simulink model "MAS_CTE"  (R2022b)
settings: Solver=ode4  StartTime=0.0  StopTime=30  FixedStep=0.01  RelTol=1e-3
(part 1 of 3)
settings Model: Creator=a1752760  LastModifiedBy=yfeih
settings SolverCC: AlgebraicLoopSolver=TrustRegion
settings DebuggingCC: UnconnectedInputMsg=warning  UnconnectedOutputMsg=warning  UnconnectedLineMsg=warning  SFMachineParentedDataDiag=warning
settings ModelReferenceCC: EnableRefExpFcnMdlSchedulingChecks=on
settings RTWCC: DLArmComputeVersion=19.05

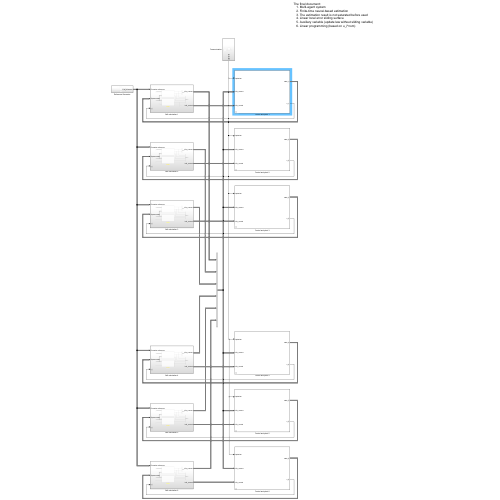
[thumbnail: Simulink's stored preview of the top-level diagram]
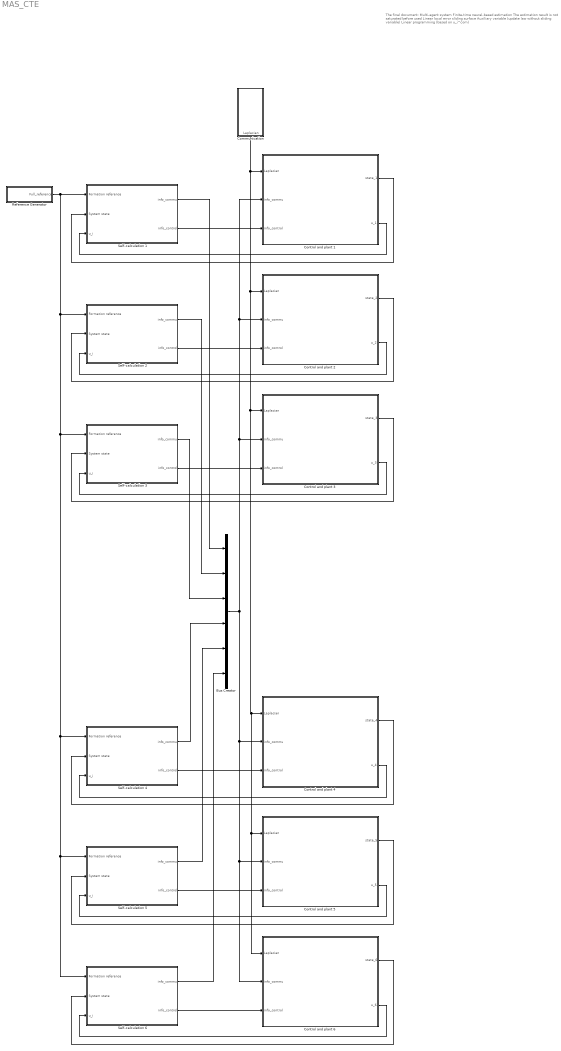
== system MAS_CTE ==
  note: The final document:
      | Multi-agent system
      | Finite-time neural-based estimation
      | The estimation result is not saturated before used
      | Linear local error sliding surface
      | Auxiliary variable (update law without sliding variable)
      | Linear programming (based on u_i^com)
  Bus Creator : BusCreator  Inputs=6
  Communication : Subsystem
  Control and plant 1 : Subsystem  mask{x_1=[3.5;1.5;pi/5], UpperLimit=0.2, LowerLimit=-0.2}
      mask prompts: x_1 "Simulink:blkprm_prompts:IntegratorInitCond"; UpperLimit "Simulink:blkprm_prompts:SaturateUpLim"; LowerLimit "Simulink:blkprm_prompts:SaturateLowLim"
      mask TypeOptions x_1: x_1/InitialCondition
      mask TypeOptions UpperLimit: Saturation/UpperLimit
      mask TypeOptions LowerLimit: Saturation/LowerLimit
      mask DialogControl x_1 Prompt: 初始条件:
      mask DialogControl UpperLimit Prompt: 上限:
      mask DialogControl LowerLimit Prompt: 下限:
  Control and plant 2 : Subsystem  mask{x_2=[-1.8;2.2;-pi/4], UpperLimit=0.2, LowerLimit=-0.2}
      mask prompts: x_2 "Simulink:blkprm_prompts:IntegratorInitCond"; UpperLimit "Simulink:blkprm_prompts:SaturateUpLim"; LowerLimit "Simulink:blkprm_prompts:SaturateLowLim"
      mask TypeOptions x_2: x_2/InitialCondition
      mask TypeOptions UpperLimit: Saturation/UpperLimit
      mask TypeOptions LowerLimit: Saturation/LowerLimit
      mask DialogControl x_2 Prompt: 初始条件:
      mask DialogControl UpperLimit Prompt: 上限:
      mask DialogControl LowerLimit Prompt: 下限:
  Control and plant 3 : Subsystem  mask{x_3=[-0.5;0.2;pi/6], UpperLimit=0.2, LowerLimit=-0.2}
      mask prompts: x_3 "Simulink:blkprm_prompts:IntegratorInitCond"; UpperLimit "Simulink:blkprm_prompts:SaturateUpLim"; LowerLimit "Simulink:blkprm_prompts:SaturateLowLim"
      mask TypeOptions x_3: x_3/InitialCondition
      mask TypeOptions UpperLimit: Saturation/UpperLimit
      mask TypeOptions LowerLimit: Saturation/LowerLimit
      mask DialogControl x_3 Prompt: 初始条件:
      mask DialogControl UpperLimit Prompt: 上限:
      mask DialogControl LowerLimit Prompt: 下限:
  Control and plant 4 : Subsystem  mask{x_4=[-1;-1.8;pi/4], UpperLimit=0.2, LowerLimit=-0.2}
      mask prompts: x_4 "Simulink:blkprm_prompts:IntegratorInitCond"; UpperLimit "Simulink:blkprm_prompts:SaturateUpLim"; LowerLimit "Simulink:blkprm_prompts:SaturateLowLim"
      mask TypeOptions x_4: x_4/InitialCondition
      mask TypeOptions UpperLimit: Saturation/UpperLimit
      mask TypeOptions LowerLimit: Saturation/LowerLimit
      mask DialogControl x_4 Prompt: 初始条件:
      mask DialogControl UpperLimit Prompt: 上限:
      mask DialogControl LowerLimit Prompt: 下限:
  Control and plant 5 : Subsystem  mask{x_5=[0.2;-1.8;-pi/4], UpperLimit=0.2, LowerLimit=-0.2}
      mask prompts: x_5 "Simulink:blkprm_prompts:IntegratorInitCond"; UpperLimit "Simulink:blkprm_prompts:SaturateUpLim"; LowerLimit "Simulink:blkprm_prompts:SaturateLowLim"
      mask TypeOptions x_5: x_5/InitialCondition
      mask TypeOptions UpperLimit: Saturation/UpperLimit
      mask TypeOptions LowerLimit: Saturation/LowerLimit
      mask DialogControl x_5 Prompt: 初始条件:
      mask DialogControl UpperLimit Prompt: 上限:
      mask DialogControl LowerLimit Prompt: 下限:
  Control and plant 6 : Subsystem  mask{x_6=[1.2;-0.8;pi/6], UpperLimit=0.2, LowerLimit=-0.2}
      mask prompts: x_6 "Simulink:blkprm_prompts:IntegratorInitCond"; UpperLimit "Simulink:blkprm_prompts:SaturateUpLim"; LowerLimit "Simulink:blkprm_prompts:SaturateLowLim"
      mask TypeOptions x_6: x_6/InitialCondition
      mask TypeOptions UpperLimit: Saturation/UpperLimit
      mask TypeOptions LowerLimit: Saturation/LowerLimit
      mask DialogControl x_6 Prompt: 初始条件:
      mask DialogControl UpperLimit Prompt: 上限:
      mask DialogControl LowerLimit Prompt: 下限:
  Reference Generator : Subsystem
  Self-calculation 1 : Subsystem
  Self-calculation 2 : Subsystem
  Self-calculation 3 : Subsystem
  Self-calculation 4 : Subsystem
  Self-calculation 5 : Subsystem
  Self-calculation 6 : Subsystem
  wires:
  Control and plant 1/1(state_1) -> Self-calculation 1/2(System state)
  Control and plant 1/2(u_1) -> Self-calculation 1/3(u_i)
  Self-calculation 1/2(info_control) -> Control and plant 1/3(info_control)
  Communication/1(Laplacian) -> Control and plant 2/1(Laplacian), Control and plant 3/1(Laplacian), Control and plant 4/1(Laplacian), Control and plant 6/1(Laplacian), Control and plant 5/1(Laplacian), Control and plant 1/1(Laplacian)
  Self-calculation 2/2(info_control) -> Control and plant 2/3(info_control)
  Control and plant 2/1(state_2) -> Self-calculation 2/2(System state)
  Control and plant 2/2(u_2) -> Self-calculation 2/3(u_i)
  Self-calculation 3/2(info_control) -> Control and plant 3/3(info_control)
  Control and plant 3/1(state_3) -> Self-calculation 3/2(System state)
  Control and plant 3/2(u_3) -> Self-calculation 3/3(u_i)
  Self-calculation 4/2(info_control) -> Control and plant 4/3(info_control)
  Control and plant 4/1(state_4) -> Self-calculation 4/2(System state)
  Control and plant 4/2(u_4) -> Self-calculation 4/3(u_i)
  Control and plant 5/1(state_5) -> Self-calculation 5/2(System state)
  Control and plant 5/2(u_5) -> Self-calculation 5/3(u_i)
  Control and plant 6/2(u_6) -> Self-calculation 6/3(u_i)
  Reference Generator/1(Full_reference) -> Self-calculation 6/1(Formation reference), Self-calculation 5/1(Formation reference), Self-calculation 4/1(Formation reference), Self-calculation 3/1(Formation reference), Self-calculation 2/1(Formation reference), Self-calculation 1/1(Formation reference)
  Control and plant 6/1(state_6) -> Self-calculation 6/2(System state)
  Self-calculation 5/2(info_control) -> Control and plant 5/3(info_control)
  Self-calculation 6/2(info_control) -> Control and plant 6/3(info_control)
  Self-calculation 1/1(info_commu) -> Bus Creator/1
  Self-calculation 2/1(info_commu) -> Bus Creator/2
  Self-calculation 3/1(info_commu) -> Bus Creator/3
  Self-calculation 4/1(info_commu) -> Bus Creator/4
  Self-calculation 5/1(info_commu) -> Bus Creator/5
  Self-calculation 6/1(info_commu) -> Bus Creator/6
  Bus Creator/1 -> Control and plant 3/2(info_commu), Control and plant 2/2(info_commu), Control and plant 1/2(info_commu), Control and plant 4/2(info_commu), Control and plant 6/2(info_commu), Control and plant 5/2(info_commu)

== system MAS_CTE/Communication ==
  Add : Sum
  Communication Topology : Constant  Value=[3,-1,0,0,-1,-1;0,1,-1,0,0,0;0,-1,2,-1,0,0;0,0,-1,2,-1,0;-1,0,0,0,1,0;0,0,0,0,-1,1]  VectorParams1D=off
  Constant : Constant  Value=2  VectorParams1D=off
  Product : Product
  Reference Feeding : Constant  Value=[1,0,0,0,0,0;0,1,0,0,0,0;0,0,1,0,0,0;0,0,0,1,0,0;0,0,0,0,1,0;0,0,0,0,0,1]  VectorParams1D=off
  Laplacian : Outport  VectorParamsAs1DForOutWhenUnconnected=off
  wires:
  Constant/1 -> Product/2
  Reference Feeding/1 -> Product/1
  Communication Topology/1 -> Add/1
  Product/1 -> Add/2
  Add/1 -> Laplacian/1

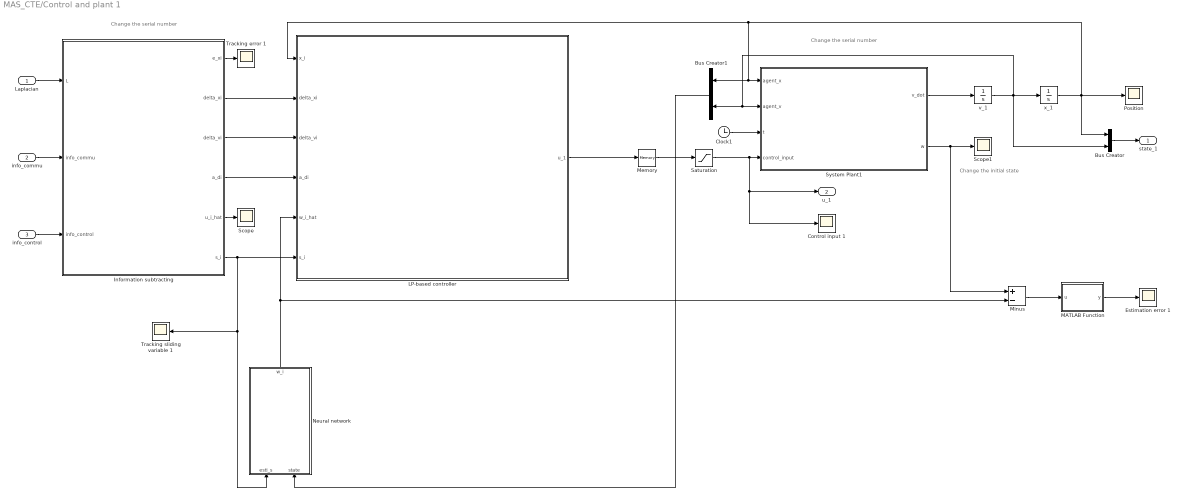
== system MAS_CTE/Control and plant 1 ==
  note: Change the serial number
  note: Change the serial number
  note: Change the initial state
  Laplacian : Inport
  info_commu : Inport  Port=2
  info_control : Inport  Port=3
  Bus Creator : BusCreator  Inputs=2
  Bus Creator1 : BusCreator  Inputs=2
  Clock1 : Clock
  Control input 1 : Scope
  Estimation error 1 : Scope
  Information subtracting : MATLAB Function  TreatAsAtomicUnit=on
  LP-based controller : Subsystem
  MATLAB Function : MATLAB Function  TreatAsAtomicUnit=on
  Memory : Memory  InitialCondition=[0;0;0]
  Minus : Sum  Inputs=+-
  Neural network : Subsystem
  Position : Scope
  Saturation : Saturate  UpperLimit=UpperLimit  LowerLimit=LowerLimit
  Scope : Scope
  Scope1 : Scope
  System Plant1 : MATLAB Function  TreatAsAtomicUnit=on
  Tracking error 1 : Scope
  Tracking sliding variable 1 : Scope
  v_1 : Integrator  InitialCondition=[0;0;0]  ContinuousStateAttributes='speed'
  x_1 : Integrator  Tag=Position_x1  InitialCondition=x_1  ContinuousStateAttributes='position'
  state_1 : Outport
  u_1 : Outport  Port=2
  wires:
  Clock1/1 -> System Plant1/3(t)
  System Plant1/1(v_dot) -> v_1/1
  v_1/1 -> Bus Creator/2, x_1/1, System Plant1/2(agent_v), Bus Creator1/2
  x_1/1 -> Bus Creator/1, Position/1, LP-based controller/1(x_i), System Plant1/1(agent_x), Bus Creator1/1
  System Plant1/2(w) -> Minus/1, Scope1/1
  Bus Creator/1 -> state_1/1
  info_commu/1 -> Information subtracting/2(info_commu)
  info_control/1 -> Information subtracting/3(info_control)
  Laplacian/1 -> Information subtracting/1(L)
  MATLAB Function/1(y) -> Estimation error 1/1
  Minus/1 -> MATLAB Function/1(u)
  Saturation/1 -> u_1/1, Control input 1/1, System Plant1/4(control_input)
  Memory/1 -> Saturation/1
  Information subtracting/1(e_xi) -> Tracking error 1/1
  LP-based controller/1(u_1) -> Memory/1
  Information subtracting/6(s_i) -> Tracking sliding variable 1/1, Neural network/1(esti_s), LP-based controller/6(s_i)
  Information subtracting/4(a_di) -> LP-based controller/4(a_di)
  Information subtracting/3(delta_vi) -> LP-based controller/3(delta_vi)
  Information subtracting/2(delta_xi) -> LP-based controller/2(delta_xi)
  Bus Creator1/1 -> Neural network/2(state)
  Information subtracting/5(u_i_hat) -> Scope/1
  Neural network/1(w_i) -> LP-based controller/5(w_i_hat), Minus/2

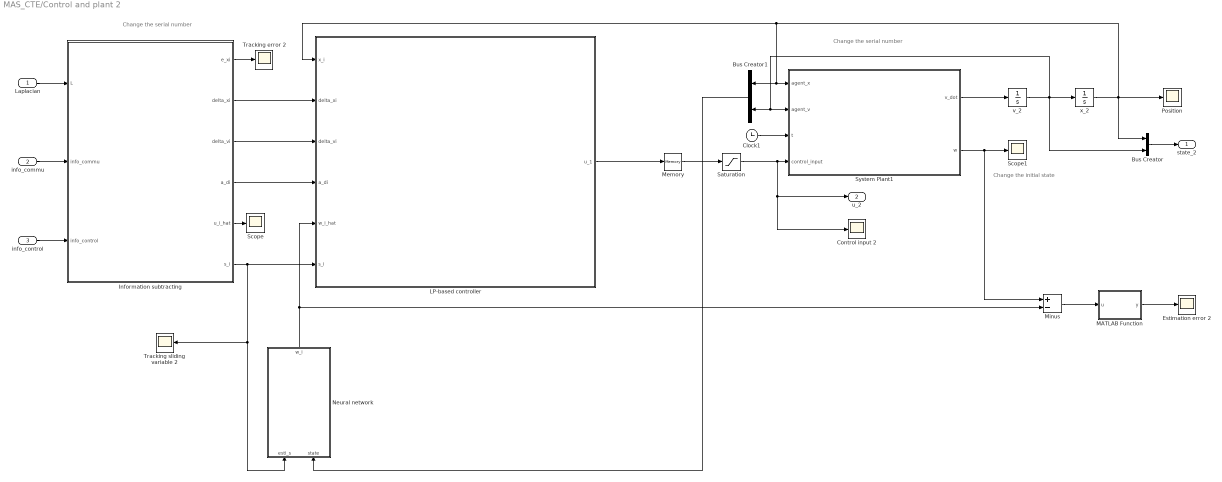
== system MAS_CTE/Control and plant 2 ==
  note: Change the serial number
  note: Change the serial number
  note: Change the initial state
  Laplacian : Inport
  info_commu : Inport  Port=2
  info_control : Inport  Port=3
  Bus Creator : BusCreator  Inputs=2
  Bus Creator1 : BusCreator  Inputs=2
  Clock1 : Clock
  Control input 2 : Scope
  Estimation error 2 : Scope
  Information subtracting : MATLAB Function  TreatAsAtomicUnit=on
  LP-based controller : Subsystem
  MATLAB Function : MATLAB Function  TreatAsAtomicUnit=on
  Memory : Memory  InitialCondition=[0;0;0]
  Minus : Sum  Inputs=+-
  Neural network : Subsystem
  Position : Scope
  Saturation : Saturate  UpperLimit=UpperLimit  LowerLimit=LowerLimit
  Scope : Scope
  Scope1 : Scope
  System Plant1 : MATLAB Function  TreatAsAtomicUnit=on
  Tracking error 2 : Scope
  Tracking sliding variable 2 : Scope
  v_2 : Integrator  InitialCondition=[0;0;0]  ContinuousStateAttributes='speed'
  x_2 : Integrator  Tag=Position_x1  InitialCondition=x_2  ContinuousStateAttributes='position'
  state_2 : Outport
  u_2 : Outport  Port=2
  wires:
  Clock1/1 -> System Plant1/3(t)
  System Plant1/1(v_dot) -> v_2/1
  v_2/1 -> Bus Creator/2, x_2/1, System Plant1/2(agent_v), Bus Creator1/2
  x_2/1 -> Bus Creator/1, Position/1, LP-based controller/1(x_i), System Plant1/1(agent_x), Bus Creator1/1
  System Plant1/2(w) -> Minus/1, Scope1/1
  Bus Creator/1 -> state_2/1
  info_commu/1 -> Information subtracting/2(info_commu)
  info_control/1 -> Information subtracting/3(info_control)
  Laplacian/1 -> Information subtracting/1(L)
  MATLAB Function/1(y) -> Estimation error 2/1
  Minus/1 -> MATLAB Function/1(u)
  Saturation/1 -> u_2/1, Control input 2/1, System Plant1/4(control_input)
  Memory/1 -> Saturation/1
  Information subtracting/1(e_xi) -> Tracking error 2/1
  LP-based controller/1(u_1) -> Memory/1
  Information subtracting/2(delta_xi) -> LP-based controller/2(delta_xi)
  Information subtracting/3(delta_vi) -> LP-based controller/3(delta_vi)
  Information subtracting/4(a_di) -> LP-based controller/4(a_di)
  Information subtracting/6(s_i) -> Tracking sliding variable 2/1, Neural network/1(esti_s), LP-based controller/6(s_i)
  Bus Creator1/1 -> Neural network/2(state)
  Information subtracting/5(u_i_hat) -> Scope/1
  Neural network/1(w_i) -> Minus/2, LP-based controller/5(w_i_hat)

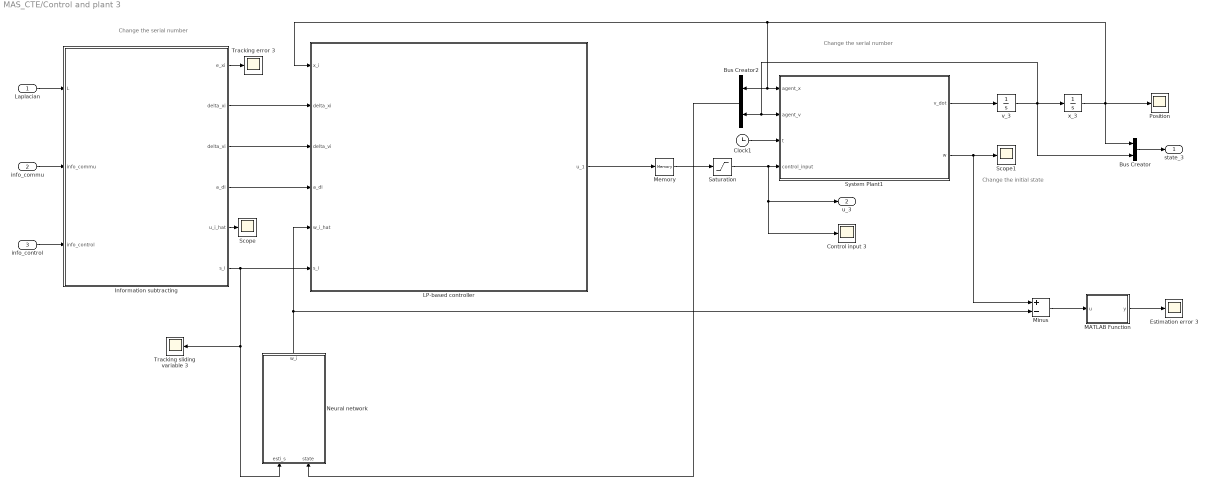
== system MAS_CTE/Control and plant 3 ==
  note: Change the serial number
  note: Change the serial number
  note: Change the initial state
  Laplacian : Inport
  info_commu : Inport  Port=2
  info_control : Inport  Port=3
  Bus Creator : BusCreator  Inputs=2
  Bus Creator2 : BusCreator  Inputs=2
  Clock1 : Clock
  Control input 3 : Scope
  Estimation error 3 : Scope
  Information subtracting : MATLAB Function  TreatAsAtomicUnit=on
  LP-based controller : Subsystem
  MATLAB Function : MATLAB Function  TreatAsAtomicUnit=on
  Memory : Memory  InitialCondition=[0;0;0]
  Minus : Sum  Inputs=+-
  Neural network : Subsystem
  Position : Scope
  Saturation : Saturate  UpperLimit=UpperLimit  LowerLimit=LowerLimit
  Scope : Scope
  Scope1 : Scope
  System Plant1 : MATLAB Function  TreatAsAtomicUnit=on
  Tracking error 3 : Scope
  Tracking sliding variable 3 : Scope
  v_3 : Integrator  InitialCondition=[0;0;0]  ContinuousStateAttributes='speed'
  x_3 : Integrator  Tag=Position_x1  InitialCondition=x_3  ContinuousStateAttributes='position'
  state_3 : Outport
  u_3 : Outport  Port=2
  wires:
  Clock1/1 -> System Plant1/3(t)
  System Plant1/1(v_dot) -> v_3/1
  v_3/1 -> Bus Creator/2, x_3/1, Bus Creator2/2, System Plant1/2(agent_v)
  x_3/1 -> Bus Creator/1, Position/1, LP-based controller/1(x_i), System Plant1/1(agent_x), Bus Creator2/1
  System Plant1/2(w) -> Minus/1, Scope1/1
  Bus Creator/1 -> state_3/1
  info_commu/1 -> Information subtracting/2(info_commu)
  info_control/1 -> Information subtracting/3(info_control)
  Laplacian/1 -> Information subtracting/1(L)
  MATLAB Function/1(y) -> Estimation error 3/1
  Minus/1 -> MATLAB Function/1(u)
  Saturation/1 -> u_3/1, Control input 3/1, System Plant1/4(control_input)
  Memory/1 -> Saturation/1
  Information subtracting/1(e_xi) -> Tracking error 3/1
  LP-based controller/1(u_1) -> Memory/1
  Information subtracting/4(a_di) -> LP-based controller/4(a_di)
  Information subtracting/3(delta_vi) -> LP-based controller/3(delta_vi)
  Information subtracting/2(delta_xi) -> LP-based controller/2(delta_xi)
  Information subtracting/5(u_i_hat) -> Scope/1
  Information subtracting/6(s_i) -> Tracking sliding variable 3/1, Neural network/1(esti_s), LP-based controller/6(s_i)
  Bus Creator2/1 -> Neural network/2(state)
  Neural network/1(w_i) -> LP-based controller/5(w_i_hat), Minus/2

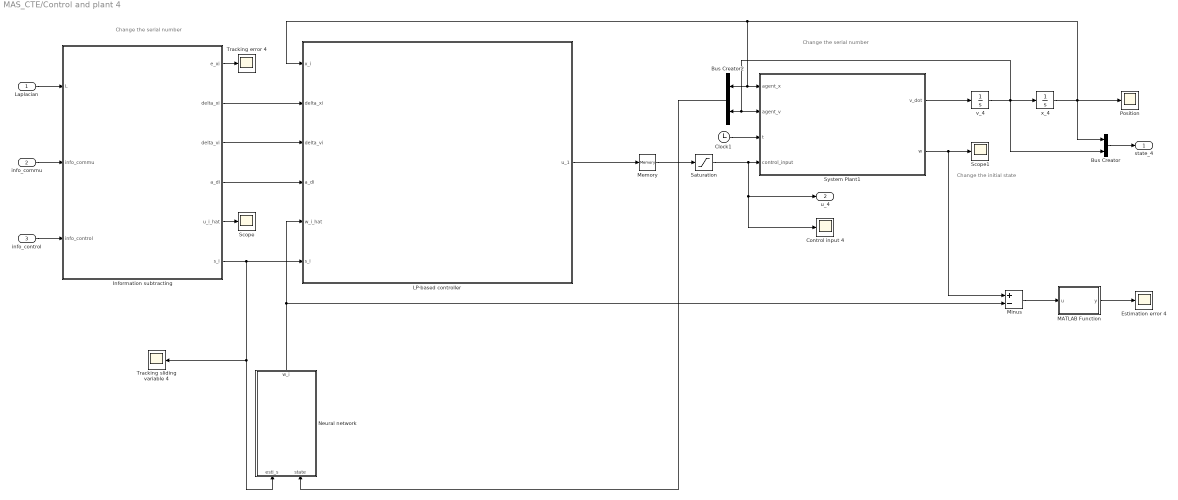
== system MAS_CTE/Control and plant 4 ==
  note: Change the serial number
  note: Change the serial number
  note: Change the initial state
  Laplacian : Inport
  info_commu : Inport  Port=2
  info_control : Inport  Port=3
  Bus Creator : BusCreator  Inputs=2
  Bus Creator2 : BusCreator  Inputs=2
  Clock1 : Clock
  Control input 4 : Scope
  Estimation error 4 : Scope
  Information subtracting : MATLAB Function  TreatAsAtomicUnit=on
  LP-based controller : Subsystem
  MATLAB Function : MATLAB Function  TreatAsAtomicUnit=on
  Memory : Memory  InitialCondition=[0;0;0]
  Minus : Sum  Inputs=+-
  Neural network : Subsystem
  Position : Scope
  Saturation : Saturate  UpperLimit=UpperLimit  LowerLimit=LowerLimit
  Scope : Scope
  Scope1 : Scope
  System Plant1 : MATLAB Function  TreatAsAtomicUnit=on
  Tracking error 4 : Scope
  Tracking sliding variable 4 : Scope
  v_4 : Integrator  InitialCondition=[0;0;0]  ContinuousStateAttributes='speed'
  x_4 : Integrator  Tag=Position_x1  InitialCondition=x_4  ContinuousStateAttributes='position'
  state_4 : Outport
  u_4 : Outport  Port=2
  wires:
  Clock1/1 -> System Plant1/3(t)
  System Plant1/1(v_dot) -> v_4/1
  v_4/1 -> Bus Creator/2, x_4/1, System Plant1/2(agent_v), Bus Creator2/2
  x_4/1 -> Bus Creator/1, Position/1, LP-based controller/1(x_i), System Plant1/1(agent_x), Bus Creator2/1
  System Plant1/2(w) -> Minus/1, Scope1/1
  Bus Creator/1 -> state_4/1
  info_commu/1 -> Information subtracting/2(info_commu)
  info_control/1 -> Information subtracting/3(info_control)
  Laplacian/1 -> Information subtracting/1(L)
  MATLAB Function/1(y) -> Estimation error 4/1
  Minus/1 -> MATLAB Function/1(u)
  Saturation/1 -> u_4/1, Control input 4/1, System Plant1/4(control_input)
  Memory/1 -> Saturation/1
  Information subtracting/1(e_xi) -> Tracking error 4/1
  LP-based controller/1(u_1) -> Memory/1
  Information subtracting/3(delta_vi) -> LP-based controller/3(delta_vi)
  Information subtracting/2(delta_xi) -> LP-based controller/2(delta_xi)
  Information subtracting/4(a_di) -> LP-based controller/4(a_di)
  Information subtracting/6(s_i) -> Tracking sliding variable 4/1, Neural network/1(esti_s), LP-based controller/6(s_i)
  Bus Creator2/1 -> Neural network/2(state)
  Neural network/1(w_i) -> Minus/2, LP-based controller/5(w_i_hat)
  Information subtracting/5(u_i_hat) -> Scope/1

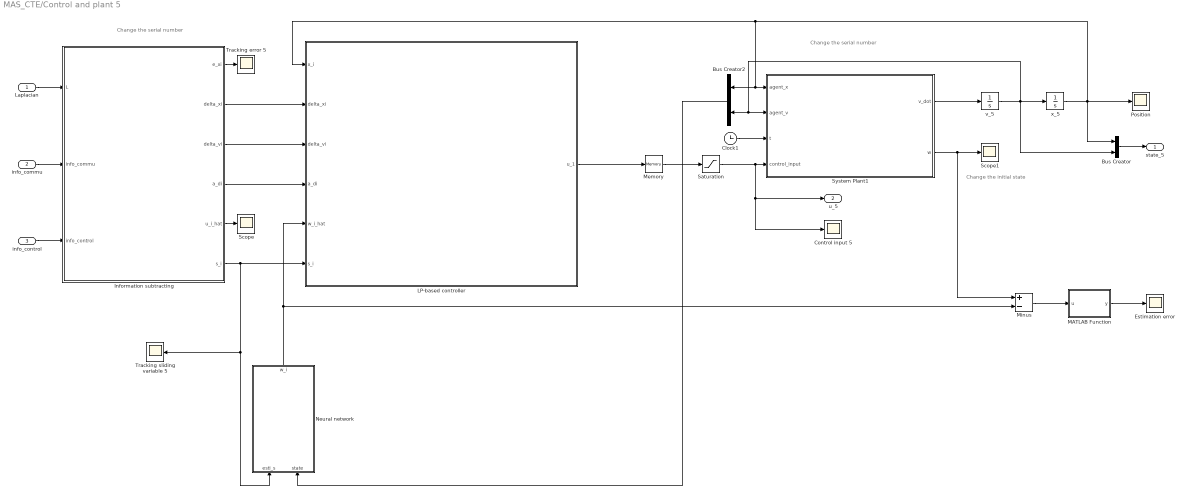
== system MAS_CTE/Control and plant 5 ==
  note: Change the serial number
  note: Change the serial number
  note: Change the initial state
  Laplacian : Inport
  info_commu : Inport  Port=2
  info_control : Inport  Port=3
  Bus Creator : BusCreator  Inputs=2
  Bus Creator2 : BusCreator  Inputs=2
  Clock1 : Clock
  Control input 5 : Scope
  Estimation error : Scope
  Information subtracting : MATLAB Function  TreatAsAtomicUnit=on
  LP-based controller : Subsystem
  MATLAB Function : MATLAB Function  TreatAsAtomicUnit=on
  Memory : Memory  InitialCondition=[0;0;0]
  Minus : Sum  Inputs=+-
  Neural network : Subsystem
  Position : Scope
  Saturation : Saturate  UpperLimit=UpperLimit  LowerLimit=LowerLimit
  Scope : Scope
  Scope1 : Scope
  System Plant1 : MATLAB Function  TreatAsAtomicUnit=on
  Tracking error 5 : Scope
  Tracking sliding variable 5 : Scope
  v_5 : Integrator  InitialCondition=[0;0;0]  ContinuousStateAttributes='speed'
  x_5 : Integrator  Tag=Position_x1  InitialCondition=x_5  ContinuousStateAttributes='position'
  state_5 : Outport
  u_5 : Outport  Port=2
  wires:
  Clock1/1 -> System Plant1/3(t)
  System Plant1/1(v_dot) -> v_5/1
  v_5/1 -> Bus Creator/2, x_5/1, System Plant1/2(agent_v), Bus Creator2/2
  x_5/1 -> Bus Creator/1, Position/1, LP-based controller/1(x_i), Bus Creator2/1, System Plant1/1(agent_x)
  System Plant1/2(w) -> Minus/1, Scope1/1
  Bus Creator/1 -> state_5/1
  info_commu/1 -> Information subtracting/2(info_commu)
  info_control/1 -> Information subtracting/3(info_control)
  Laplacian/1 -> Information subtracting/1(L)
  MATLAB Function/1(y) -> Estimation error/1
  Minus/1 -> MATLAB Function/1(u)
  Saturation/1 -> u_5/1, Control input 5/1, System Plant1/4(control_input)
  Memory/1 -> Saturation/1
  Information subtracting/1(e_xi) -> Tracking error 5/1
  LP-based controller/1(u_1) -> Memory/1
  Information subtracting/3(delta_vi) -> LP-based controller/3(delta_vi)
  Information subtracting/2(delta_xi) -> LP-based controller/2(delta_xi)
  Information subtracting/4(a_di) -> LP-based controller/4(a_di)
  Information subtracting/6(s_i) -> Tracking sliding variable 5/1, Neural network/1(esti_s), LP-based controller/6(s_i)
  Bus Creator2/1 -> Neural network/2(state)
  Information subtracting/5(u_i_hat) -> Scope/1
  Neural network/1(w_i) -> Minus/2, LP-based controller/5(w_i_hat)

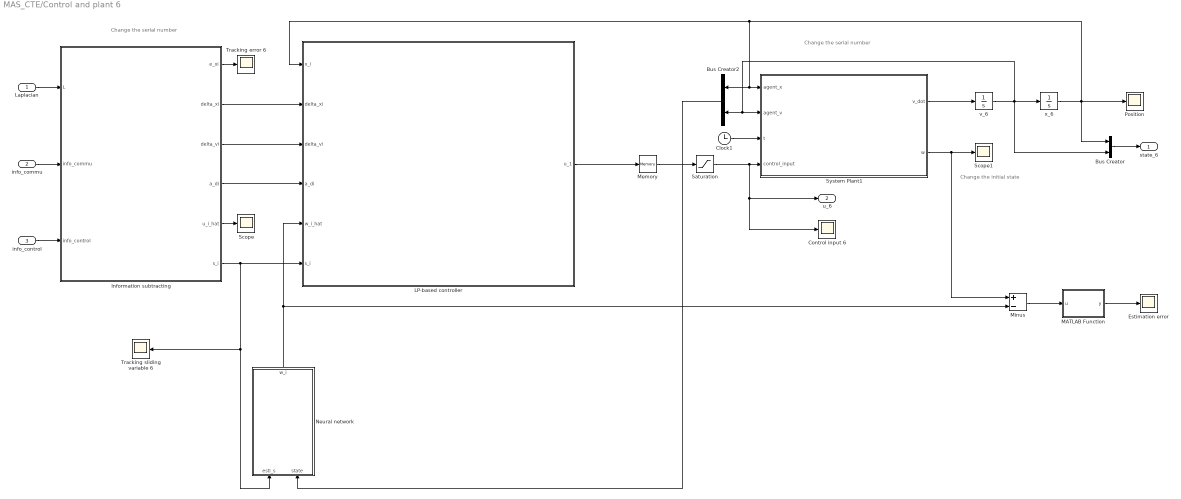
== system MAS_CTE/Control and plant 6 ==
  note: Change the serial number
  note: Change the serial number
  note: Change the initial state
  Laplacian : Inport
  info_commu : Inport  Port=2
  info_control : Inport  Port=3
  Bus Creator : BusCreator  Inputs=2
  Bus Creator2 : BusCreator  Inputs=2
  Clock1 : Clock
  Control input 6 : Scope
  Estimation error : Scope
  Information subtracting : MATLAB Function  TreatAsAtomicUnit=on
  LP-based controller : Subsystem
  MATLAB Function : MATLAB Function  TreatAsAtomicUnit=on
  Memory : Memory  InitialCondition=[0;0;0]
  Minus : Sum  Inputs=+-
  Neural network : Subsystem
  Position : Scope
  Saturation : Saturate  UpperLimit=UpperLimit  LowerLimit=LowerLimit
  Scope : Scope
  Scope1 : Scope
  System Plant1 : MATLAB Function  TreatAsAtomicUnit=on
  Tracking error 6 : Scope
  Tracking sliding variable 6 : Scope
  v_6 : Integrator  InitialCondition=[0;0;0]  ContinuousStateAttributes='speed'
  x_6 : Integrator  Tag=Position_x1  InitialCondition=x_6  ContinuousStateAttributes='position'
  state_6 : Outport
  u_6 : Outport  Port=2
  wires:
  Clock1/1 -> System Plant1/3(t)
  System Plant1/1(v_dot) -> v_6/1
  v_6/1 -> Bus Creator/2, x_6/1, System Plant1/2(agent_v), Bus Creator2/2
  x_6/1 -> Bus Creator/1, Position/1, LP-based controller/1(x_i), System Plant1/1(agent_x), Bus Creator2/1
  System Plant1/2(w) -> Minus/1, Scope1/1
  Bus Creator/1 -> state_6/1
  info_commu/1 -> Information subtracting/2(info_commu)
  info_control/1 -> Information subtracting/3(info_control)
  Laplacian/1 -> Information subtracting/1(L)
  MATLAB Function/1(y) -> Estimation error/1
  Minus/1 -> MATLAB Function/1(u)
  Saturation/1 -> u_6/1, Control input 6/1, System Plant1/4(control_input)
  Memory/1 -> Saturation/1
  Information subtracting/1(e_xi) -> Tracking error 6/1
  LP-based controller/1(u_1) -> Memory/1
  Information subtracting/2(delta_xi) -> LP-based controller/2(delta_xi)
  Information subtracting/3(delta_vi) -> LP-based controller/3(delta_vi)
  Information subtracting/4(a_di) -> LP-based controller/4(a_di)
  Information subtracting/6(s_i) -> Tracking sliding variable 6/1, Neural network/1(esti_s), LP-based controller/6(s_i)
  Bus Creator2/1 -> Neural network/2(state)
  Neural network/1(w_i) -> Minus/2, LP-based controller/5(w_i_hat)
  Information subtracting/5(u_i_hat) -> Scope/1

== system MAS_CTE/Reference Generator ==
  Acceleration Reference : MATLAB Function  TreatAsAtomicUnit=on
  Bus Creator : BusCreator  Inputs=3
  Centre acceleration : Scope
  Centre position : Scope
  Centre velocity : Scope
  Clock : Clock
  Position Reference : MATLAB Function  TreatAsAtomicUnit=on
  Position_ref : Scope
  Velocity Reference : MATLAB Function  TreatAsAtomicUnit=on
  Full_reference : Outport  VectorParamsAs1DForOutWhenUnconnected=off
  wires:
  Clock/1 -> Velocity Reference/1(t), Acceleration Reference/1(t), Position Reference/1(t)
  Position Reference/1(x_d) -> Bus Creator/1, Position_ref/1
  Position Reference/2(centre) -> Centre position/1
  Velocity Reference/2(centre) -> Centre velocity/1
  Acceleration Reference/2(centre) -> Centre acceleration/1
  Velocity Reference/1(v_d) -> Bus Creator/2
  Acceleration Reference/1(a_d) -> Bus Creator/3
  Bus Creator/1 -> Full_reference/1

== system MAS_CTE/Self-calculation 1 ==
  note: Change the serial number
  Formation reference : Inport
  System state : Inport  Port=2
  u_i : Inport  Port=3
  Bus Creator : BusCreator  Inputs=4
  Bus Creator1 : BusCreator  Inputs=2
  E_1 : Scope
  Observer : Subsystem  mask{InitialCondition=[3.5;1.5;pi/5]}
      mask prompts: InitialCondition "Simulink:blkprm_prompts:IntegratorInitCond"
      mask TypeOptions InitialCondition: virtual_pos/InitialCondition
      mask DialogControl InitialCondition Prompt: 初始条件:
  Tracking error calculation : Subsystem
  info_commu : Outport
  info_control : Outport  Port=2
  wires:
  Formation reference/1 -> Tracking error calculation/1(ref)
  System state/1 -> Tracking error calculation/2(state), Observer/1(state)
  Tracking error calculation/1(delta_xi) -> Bus Creator/1, Bus Creator1/1
  Tracking error calculation/2(delta_vi) -> Bus Creator/2, Bus Creator1/2
  Tracking error calculation/3(a_d) -> Bus Creator/3
  Bus Creator1/1 -> info_commu/1
  Bus Creator/1 -> info_control/1
  u_i/1 -> Observer/2(u_i)
  Observer/1(E_i) -> E_1/1, Bus Creator/4

== system MAS_CTE/Self-calculation 2 ==
  note: Change the serial number
  Formation reference : Inport
  System state : Inport  Port=2
  u_i : Inport  Port=3
  Bus Creator : BusCreator  Inputs=4
  Bus Creator1 : BusCreator  Inputs=2
  Observer : Subsystem  mask{InitialCondition=[-1.8;2.2;-pi/4]}
      mask prompts: InitialCondition "Simulink:blkprm_prompts:IntegratorInitCond"
      mask TypeOptions InitialCondition: virtual_pos/InitialCondition
      mask DialogControl InitialCondition Prompt: 初始条件:
  Tracking error calculation : Subsystem
  info_commu : Outport
  info_control : Outport  Port=2
  wires:
  Formation reference/1 -> Tracking error calculation/1(ref)
  System state/1 -> Observer/1(state), Tracking error calculation/2(state)
  Tracking error calculation/1(delta_xi) -> Bus Creator/1, Bus Creator1/1
  Tracking error calculation/2(delta_vi) -> Bus Creator/2, Bus Creator1/2
  Tracking error calculation/3(a_d) -> Bus Creator/3
  Observer/1(E_i) -> Bus Creator/4
  Bus Creator1/1 -> info_commu/1
  Bus Creator/1 -> info_control/1
  u_i/1 -> Observer/2(u_i)

== system MAS_CTE/Self-calculation 3 ==
  note: Change the serial number
  Formation reference : Inport
  System state : Inport  Port=2
  u_i : Inport  Port=3
  Bus Creator : BusCreator  Inputs=4
  Bus Creator1 : BusCreator  Inputs=2
  Observer : Subsystem  mask{InitialCondition=[-0.5;0.2;pi/6]}
      mask prompts: InitialCondition "Simulink:blkprm_prompts:IntegratorInitCond"
      mask TypeOptions InitialCondition: virtual_pos/InitialCondition
      mask DialogControl InitialCondition Prompt: 初始条件:
  Tracking error calculation : Subsystem
  info_commu : Outport
  info_control : Outport  Port=2
  wires:
  Formation reference/1 -> Tracking error calculation/1(ref)
  System state/1 -> Observer/1(state), Tracking error calculation/2(state)
  Tracking error calculation/1(delta_xi) -> Bus Creator/1, Bus Creator1/1
  Tracking error calculation/2(delta_vi) -> Bus Creator/2, Bus Creator1/2
  Tracking error calculation/3(a_d) -> Bus Creator/3
  Observer/1(E_i) -> Bus Creator/4
  Bus Creator1/1 -> info_commu/1
  Bus Creator/1 -> info_control/1
  u_i/1 -> Observer/2(u_i)

== system MAS_CTE/Self-calculation 4 ==
  note: Change the serial number
  Formation reference : Inport
  System state : Inport  Port=2
  u_i : Inport  Port=3
  Bus Creator : BusCreator  Inputs=4
  Bus Creator1 : BusCreator  Inputs=2
  Observer : Subsystem  mask{InitialCondition=[-1;-1.8;pi/4]}
      mask prompts: InitialCondition "Simulink:blkprm_prompts:IntegratorInitCond"
      mask TypeOptions InitialCondition: virtual_pos/InitialCondition
      mask DialogControl InitialCondition Prompt: 初始条件:
  Tracking error calculation : Subsystem
  info_commu : Outport
  info_control : Outport  Port=2
  wires:
  Formation reference/1 -> Tracking error calculation/1(ref)
  System state/1 -> Observer/1(state), Tracking error calculation/2(state)
  Tracking error calculation/1(delta_xi) -> Bus Creator/1, Bus Creator1/1
  Tracking error calculation/2(delta_vi) -> Bus Creator/2, Bus Creator1/2
  Tracking error calculation/3(a_d) -> Bus Creator/3
  Observer/1(E_i) -> Bus Creator/4
  Bus Creator1/1 -> info_commu/1
  Bus Creator/1 -> info_control/1
  u_i/1 -> Observer/2(u_i)

== system MAS_CTE/Self-calculation 5 ==
  note: Change the serial number
  Formation reference : Inport
  System state : Inport  Port=2
  u_i : Inport  Port=3
  Bus Creator : BusCreator  Inputs=4
  Bus Creator1 : BusCreator  Inputs=2
  Observer : Subsystem  mask{InitialCondition=[0.2;-1.8;-pi/4]}
      mask prompts: InitialCondition "Simulink:blkprm_prompts:IntegratorInitCond"
      mask TypeOptions InitialCondition: virtual_pos/InitialCondition
      mask DialogControl InitialCondition Prompt: 初始条件:
  Tracking error calculation : Subsystem
  info_commu : Outport
  info_control : Outport  Port=2
  wires:
  Formation reference/1 -> Tracking error calculation/1(ref)
  System state/1 -> Observer/1(state), Tracking error calculation/2(state)
  Tracking error calculation/1(delta_xi) -> Bus Creator/1, Bus Creator1/1
  Tracking error calculation/2(delta_vi) -> Bus Creator/2, Bus Creator1/2
  Tracking error calculation/3(a_d) -> Bus Creator/3
  Observer/1(E_i) -> Bus Creator/4
  Bus Creator1/1 -> info_commu/1
  Bus Creator/1 -> info_control/1
  u_i/1 -> Observer/2(u_i)

== system MAS_CTE/Self-calculation 6 ==
  note: Change the serial number
  Formation reference : Inport
  System state : Inport  Port=2
  u_i : Inport  Port=3
  Bus Creator : BusCreator  Inputs=4
  Bus Creator1 : BusCreator  Inputs=2
  Observer : Subsystem  mask{InitialCondition=[1.2;-0.8;pi/6]}
      mask prompts: InitialCondition "Simulink:blkprm_prompts:IntegratorInitCond"
      mask TypeOptions InitialCondition: virtual_pos/InitialCondition
      mask DialogControl InitialCondition Prompt: 初始条件:
  Tracking error calculation : Subsystem
  info_commu : Outport
  info_control : Outport  Port=2
  wires:
  Formation reference/1 -> Tracking error calculation/1(ref)
  System state/1 -> Observer/1(state), Tracking error calculation/2(state)
  Tracking error calculation/1(delta_xi) -> Bus Creator/1, Bus Creator1/1
  Tracking error calculation/2(delta_vi) -> Bus Creator/2, Bus Creator1/2
  Tracking error calculation/3(a_d) -> Bus Creator/3
  Observer/1(E_i) -> Bus Creator/4
  Bus Creator1/1 -> info_commu/1
  Bus Creator/1 -> info_control/1
  u_i/1 -> Observer/2(u_i)

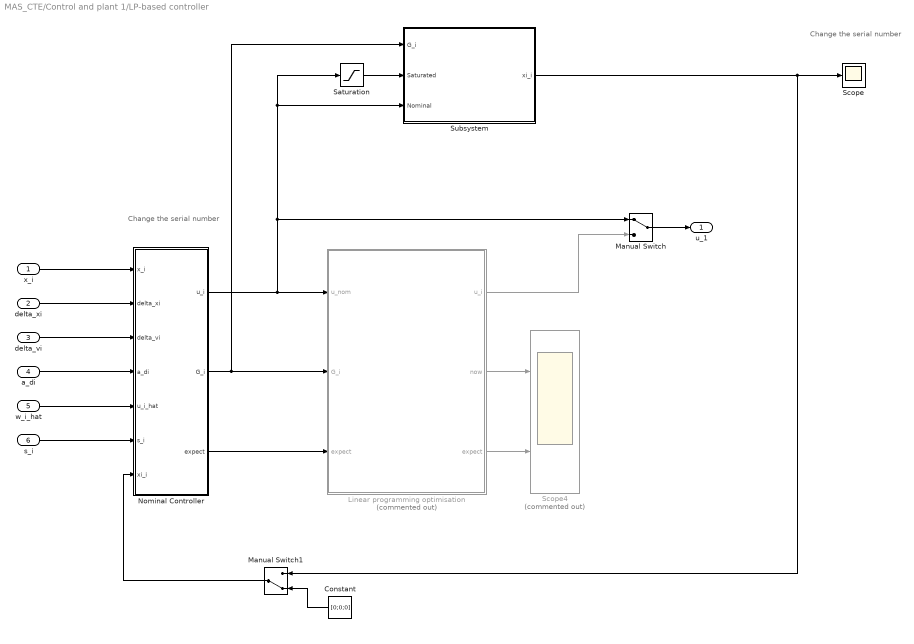
== system MAS_CTE/Control and plant 1/LP-based controller ==
  note: Change the serial number
  note: Change the serial number
  x_i : Inport
  delta_xi : Inport  Port=2
  delta_vi : Inport  Port=3
  a_di : Inport  Port=4
  w_i_hat : Inport  Port=5
  s_i : Inport  Port=6
  Constant : Constant  Value=[0;0;0]
  Linear programming optimisation : MATLAB Function  Commented=on  TreatAsAtomicUnit=on
  Manual Switch : ManualSwitch
  Manual Switch1 : ManualSwitch  CurrentSetting=0
  Nominal Controller : MATLAB Function  TreatAsAtomicUnit=on
  Saturation : Saturate  UpperLimit=UpperLimit  LowerLimit=LowerLimit
  Scope : Scope
  Scope4 : Scope  Commented=on  NumInputPorts=2
  Subsystem : Subsystem
  u_1 : Outport
  wires:
  Nominal Controller/2(G_i) -> Subsystem/1(G_i), Linear programming optimisation/2(G_i)
  Linear programming optimisation/1(u_i) -> Manual Switch/2
  Nominal Controller/3(expect) -> Linear programming optimisation/3("expect ")
  Linear programming optimisation/2(now) -> Scope4/1
  Linear programming optimisation/3(expect) -> Scope4/2
  Nominal Controller/1(u_i) -> Subsystem/3(Nominal), Saturation/1, Manual Switch/1, Linear programming optimisation/1(u_nom)
  x_i/1 -> Nominal Controller/1(x_i)
  delta_xi/1 -> Nominal Controller/2(delta_xi)
  delta_vi/1 -> Nominal Controller/3(delta_vi)
  a_di/1 -> Nominal Controller/4(a_di)
  w_i_hat/1 -> Nominal Controller/5(u_i_hat)
  s_i/1 -> Nominal Controller/6(s_i)
  Saturation/1 -> Subsystem/2(Saturated)
  Manual Switch/1 -> u_1/1
  Subsystem/1(xi_i) -> Manual Switch1/1, Scope/1
  Constant/1 -> Manual Switch1/2
  Manual Switch1/1 -> Nominal Controller/7(xi_i)

== system MAS_CTE/Control and plant 1/Neural network ==
  esti_s : Inport
  state : Inport  Port=2
  Hyperbolic : MATLAB Function  TreatAsAtomicUnit=on
  Manual Switch : ManualSwitch
  Neural network output : MATLAB Function  TreatAsAtomicUnit=on
  Update of neural weight : MATLAB Function  TreatAsAtomicUnit=on
  Weight initialisation : MATLAB Function  TreatAsAtomicUnit=on
  Weight update : Integrator  InitialConditionSource=external
  w_i : Outport
  wires:
  Update of neural weight/1(W_dot) -> Weight update/1
  esti_s/1 -> Update of neural weight/2(esti_s)
  Neural network output/1(w_i) -> w_i/1
  Weight initialisation/1(W_0) -> Weight update/2
  Weight update/1 -> Update of neural weight/3(W), Neural network output/2(W)
  Manual Switch/1 -> Neural network output/1(phi_net), Update of neural weight/1(phi_net)
  Hyperbolic/1(output) -> Manual Switch/1
  state/1 -> Hyperbolic/1(input), Manual Switch/2

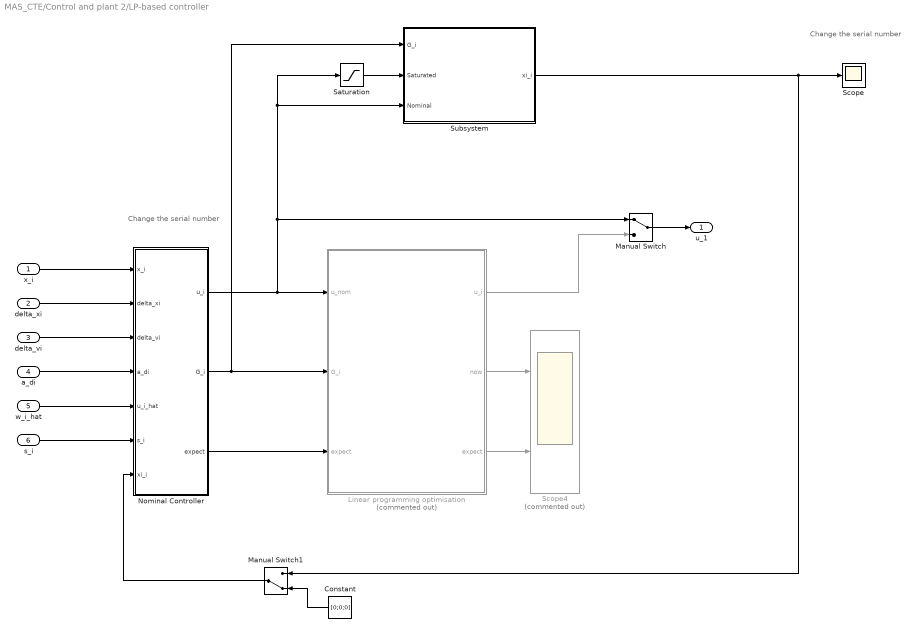
== system MAS_CTE/Control and plant 2/LP-based controller ==
  note: Change the serial number
  note: Change the serial number
  x_i : Inport
  delta_xi : Inport  Port=2
  delta_vi : Inport  Port=3
  a_di : Inport  Port=4
  w_i_hat : Inport  Port=5
  s_i : Inport  Port=6
  Constant : Constant  Value=[0;0;0]
  Linear programming optimisation : MATLAB Function  Commented=on  TreatAsAtomicUnit=on
  Manual Switch : ManualSwitch
  Manual Switch1 : ManualSwitch  CurrentSetting=0
  Nominal Controller : MATLAB Function  TreatAsAtomicUnit=on
  Saturation : Saturate  UpperLimit=UpperLimit  LowerLimit=LowerLimit
  Scope : Scope
  Scope4 : Scope  Commented=on  NumInputPorts=2
  Subsystem : Subsystem
  u_1 : Outport
  wires:
  Nominal Controller/2(G_i) -> Subsystem/1(G_i), Linear programming optimisation/2(G_i)
  Linear programming optimisation/1(u_i) -> Manual Switch/2
  Nominal Controller/3(expect) -> Linear programming optimisation/3("expect ")
  Linear programming optimisation/2(now) -> Scope4/1
  Linear programming optimisation/3(expect) -> Scope4/2
  Nominal Controller/1(u_i) -> Subsystem/3(Nominal), Saturation/1, Manual Switch/1, Linear programming optimisation/1(u_nom)
  x_i/1 -> Nominal Controller/1(x_i)
  delta_xi/1 -> Nominal Controller/2(delta_xi)
  delta_vi/1 -> Nominal Controller/3(delta_vi)
  a_di/1 -> Nominal Controller/4(a_di)
  w_i_hat/1 -> Nominal Controller/5(u_i_hat)
  s_i/1 -> Nominal Controller/6(s_i)
  Saturation/1 -> Subsystem/2(Saturated)
  Manual Switch/1 -> u_1/1
  Subsystem/1(xi_i) -> Manual Switch1/1, Scope/1
  Constant/1 -> Manual Switch1/2
  Manual Switch1/1 -> Nominal Controller/7(xi_i)

== system MAS_CTE/Control and plant 2/Neural network ==
  esti_s : Inport
  state : Inport  Port=2
  Hyperbolic : MATLAB Function  TreatAsAtomicUnit=on
  Manual Switch : ManualSwitch
  Neural network output : MATLAB Function  TreatAsAtomicUnit=on
  Update of neural weight : MATLAB Function  TreatAsAtomicUnit=on
  Weight initialisation : MATLAB Function  TreatAsAtomicUnit=on
  Weight update : Integrator  InitialConditionSource=external
  w_i : Outport
  wires:
  Update of neural weight/1(W_dot) -> Weight update/1
  esti_s/1 -> Update of neural weight/2(esti_s)
  Neural network output/1(w_i) -> w_i/1
  Weight initialisation/1(W_0) -> Weight update/2
  Weight update/1 -> Update of neural weight/3(W), Neural network output/2(W)
  Manual Switch/1 -> Neural network output/1(phi_net), Update of neural weight/1(phi_net)
  Hyperbolic/1(output) -> Manual Switch/1
  state/1 -> Hyperbolic/1(input), Manual Switch/2

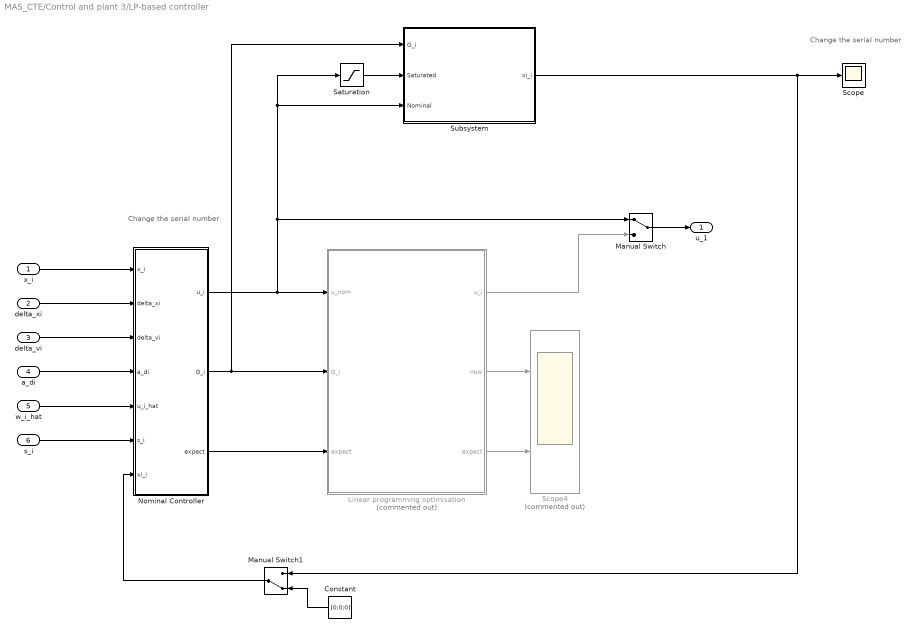
== system MAS_CTE/Control and plant 3/LP-based controller ==
  note: Change the serial number
  note: Change the serial number
  x_i : Inport
  delta_xi : Inport  Port=2
  delta_vi : Inport  Port=3
  a_di : Inport  Port=4
  w_i_hat : Inport  Port=5
  s_i : Inport  Port=6
  Constant : Constant  Value=[0;0;0]
  Linear programming optimisation : MATLAB Function  Commented=on  TreatAsAtomicUnit=on
  Manual Switch : ManualSwitch
  Manual Switch1 : ManualSwitch  CurrentSetting=0
  Nominal Controller : MATLAB Function  TreatAsAtomicUnit=on
  Saturation : Saturate  UpperLimit=UpperLimit  LowerLimit=LowerLimit
  Scope : Scope
  Scope4 : Scope  Commented=on  NumInputPorts=2
  Subsystem : Subsystem
  u_1 : Outport
  wires:
  Nominal Controller/2(G_i) -> Subsystem/1(G_i), Linear programming optimisation/2(G_i)
  Linear programming optimisation/1(u_i) -> Manual Switch/2
  Nominal Controller/3(expect) -> Linear programming optimisation/3("expect ")
  Linear programming optimisation/2(now) -> Scope4/1
  Linear programming optimisation/3(expect) -> Scope4/2
  Nominal Controller/1(u_i) -> Subsystem/3(Nominal), Saturation/1, Manual Switch/1, Linear programming optimisation/1(u_nom)
  x_i/1 -> Nominal Controller/1(x_i)
  delta_xi/1 -> Nominal Controller/2(delta_xi)
  delta_vi/1 -> Nominal Controller/3(delta_vi)
  a_di/1 -> Nominal Controller/4(a_di)
  w_i_hat/1 -> Nominal Controller/5(u_i_hat)
  s_i/1 -> Nominal Controller/6(s_i)
  Saturation/1 -> Subsystem/2(Saturated)
  Manual Switch/1 -> u_1/1
  Subsystem/1(xi_i) -> Manual Switch1/1, Scope/1
  Constant/1 -> Manual Switch1/2
  Manual Switch1/1 -> Nominal Controller/7(xi_i)

== system MAS_CTE/Control and plant 3/Neural network ==
  esti_s : Inport
  state : Inport  Port=2
  Hyperbolic : MATLAB Function  TreatAsAtomicUnit=on
  Manual Switch : ManualSwitch
  Neural network output : MATLAB Function  TreatAsAtomicUnit=on
  Update of neural weight : MATLAB Function  TreatAsAtomicUnit=on
  Weight initialisation : MATLAB Function  TreatAsAtomicUnit=on
  Weight update : Integrator  InitialConditionSource=external
  w_i : Outport
  wires:
  Update of neural weight/1(W_dot) -> Weight update/1
  esti_s/1 -> Update of neural weight/2(esti_s)
  Neural network output/1(w_i) -> w_i/1
  Weight initialisation/1(W_0) -> Weight update/2
  Weight update/1 -> Update of neural weight/3(W), Neural network output/2(W)
  Manual Switch/1 -> Neural network output/1(phi_net), Update of neural weight/1(phi_net)
  Hyperbolic/1(output) -> Manual Switch/1
  state/1 -> Hyperbolic/1(input), Manual Switch/2

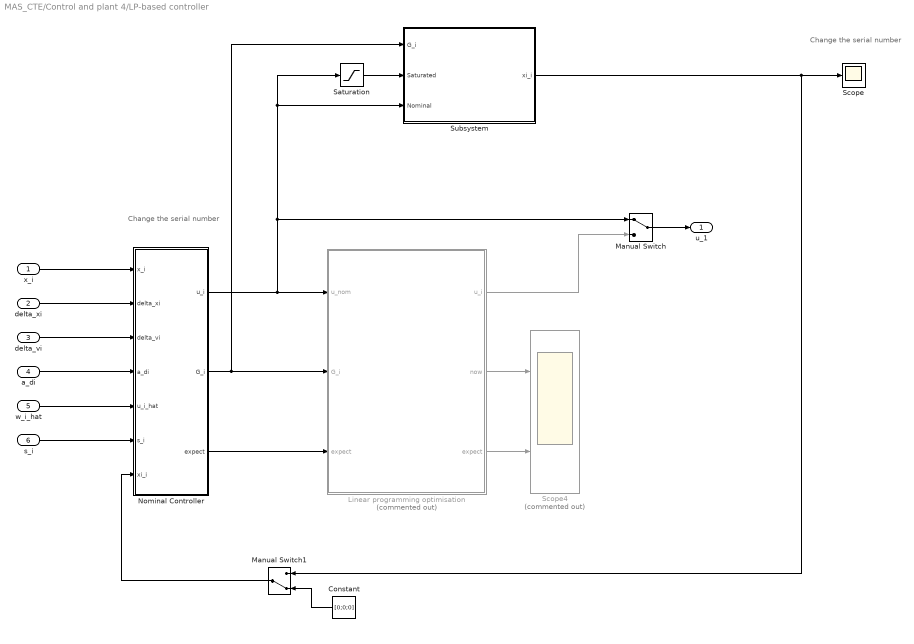
== system MAS_CTE/Control and plant 4/LP-based controller ==
  note: Change the serial number
  note: Change the serial number
  x_i : Inport
  delta_xi : Inport  Port=2
  delta_vi : Inport  Port=3
  a_di : Inport  Port=4
  w_i_hat : Inport  Port=5
  s_i : Inport  Port=6
  Constant : Constant  Value=[0;0;0]
  Linear programming optimisation : MATLAB Function  Commented=on  TreatAsAtomicUnit=on
  Manual Switch : ManualSwitch
  Manual Switch1 : ManualSwitch  CurrentSetting=0
  Nominal Controller : MATLAB Function  TreatAsAtomicUnit=on
  Saturation : Saturate  UpperLimit=UpperLimit  LowerLimit=LowerLimit
  Scope : Scope
  Scope4 : Scope  Commented=on  NumInputPorts=2
  Subsystem : Subsystem
  u_1 : Outport
  wires:
  Nominal Controller/2(G_i) -> Subsystem/1(G_i), Linear programming optimisation/2(G_i)
  Linear programming optimisation/1(u_i) -> Manual Switch/2
  Nominal Controller/3(expect) -> Linear programming optimisation/3("expect ")
  Linear programming optimisation/2(now) -> Scope4/1
  Linear programming optimisation/3(expect) -> Scope4/2
  Nominal Controller/1(u_i) -> Subsystem/3(Nominal), Saturation/1, Manual Switch/1, Linear programming optimisation/1(u_nom)
  x_i/1 -> Nominal Controller/1(x_i)
  delta_xi/1 -> Nominal Controller/2(delta_xi)
  delta_vi/1 -> Nominal Controller/3(delta_vi)
  a_di/1 -> Nominal Controller/4(a_di)
  w_i_hat/1 -> Nominal Controller/5(u_i_hat)
  s_i/1 -> Nominal Controller/6(s_i)
  Saturation/1 -> Subsystem/2(Saturated)
  Manual Switch/1 -> u_1/1
  Subsystem/1(xi_i) -> Manual Switch1/1, Scope/1
  Constant/1 -> Manual Switch1/2
  Manual Switch1/1 -> Nominal Controller/7(xi_i)

== system MAS_CTE/Control and plant 4/Neural network ==
  esti_s : Inport
  state : Inport  Port=2
  Hyperbolic : MATLAB Function  TreatAsAtomicUnit=on
  Manual Switch : ManualSwitch
  Neural network output : MATLAB Function  TreatAsAtomicUnit=on
  Update of neural weight : MATLAB Function  TreatAsAtomicUnit=on
  Weight initialisation : MATLAB Function  TreatAsAtomicUnit=on
  Weight update : Integrator  InitialConditionSource=external
  w_i : Outport
  wires:
  Update of neural weight/1(W_dot) -> Weight update/1
  esti_s/1 -> Update of neural weight/2(esti_s)
  Neural network output/1(w_i) -> w_i/1
  Weight initialisation/1(W_0) -> Weight update/2
  Weight update/1 -> Update of neural weight/3(W), Neural network output/2(W)
  Manual Switch/1 -> Neural network output/1(phi_net), Update of neural weight/1(phi_net)
  Hyperbolic/1(output) -> Manual Switch/1
  state/1 -> Hyperbolic/1(input), Manual Switch/2

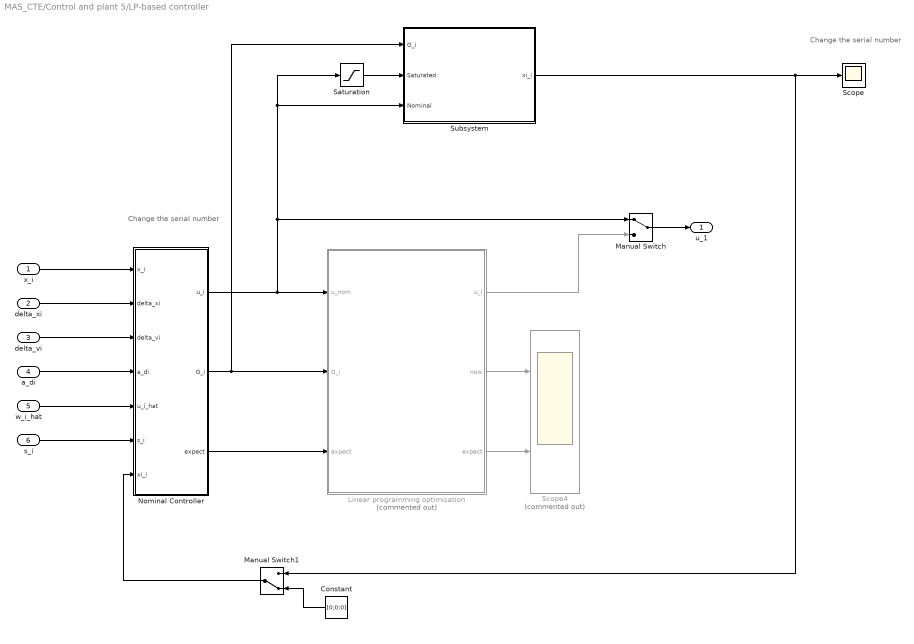
== system MAS_CTE/Control and plant 5/LP-based controller ==
  note: Change the serial number
  note: Change the serial number
  x_i : Inport
  delta_xi : Inport  Port=2
  delta_vi : Inport  Port=3
  a_di : Inport  Port=4
  w_i_hat : Inport  Port=5
  s_i : Inport  Port=6
  Constant : Constant  Value=[0;0;0]
  Linear programming optimisation : MATLAB Function  Commented=on  TreatAsAtomicUnit=on
  Manual Switch : ManualSwitch
  Manual Switch1 : ManualSwitch  CurrentSetting=0
  Nominal Controller : MATLAB Function  TreatAsAtomicUnit=on
  Saturation : Saturate  UpperLimit=UpperLimit  LowerLimit=LowerLimit
  Scope : Scope
  Scope4 : Scope  Commented=on  NumInputPorts=2
  Subsystem : Subsystem
  u_1 : Outport
  wires:
  Nominal Controller/2(G_i) -> Subsystem/1(G_i), Linear programming optimisation/2(G_i)
  Linear programming optimisation/1(u_i) -> Manual Switch/2
  Nominal Controller/3(expect) -> Linear programming optimisation/3("expect ")
  Linear programming optimisation/2(now) -> Scope4/1
  Linear programming optimisation/3(expect) -> Scope4/2
  Nominal Controller/1(u_i) -> Subsystem/3(Nominal), Saturation/1, Manual Switch/1, Linear programming optimisation/1(u_nom)
  x_i/1 -> Nominal Controller/1(x_i)
  delta_xi/1 -> Nominal Controller/2(delta_xi)
  delta_vi/1 -> Nominal Controller/3(delta_vi)
  a_di/1 -> Nominal Controller/4(a_di)
  w_i_hat/1 -> Nominal Controller/5(u_i_hat)
  s_i/1 -> Nominal Controller/6(s_i)
  Saturation/1 -> Subsystem/2(Saturated)
  Manual Switch/1 -> u_1/1
  Subsystem/1(xi_i) -> Manual Switch1/1, Scope/1
  Constant/1 -> Manual Switch1/2
  Manual Switch1/1 -> Nominal Controller/7(xi_i)

== system MAS_CTE/Control and plant 5/Neural network ==
  esti_s : Inport
  state : Inport  Port=2
  Hyperbolic : MATLAB Function  TreatAsAtomicUnit=on
  Manual Switch : ManualSwitch
  Neural network output : MATLAB Function  TreatAsAtomicUnit=on
  Update of neural weight : MATLAB Function  TreatAsAtomicUnit=on
  Weight initialisation : MATLAB Function  TreatAsAtomicUnit=on
  Weight update : Integrator  InitialConditionSource=external
  w_i : Outport
  wires:
  Update of neural weight/1(W_dot) -> Weight update/1
  esti_s/1 -> Update of neural weight/2(esti_s)
  Neural network output/1(w_i) -> w_i/1
  Weight initialisation/1(W_0) -> Weight update/2
  Weight update/1 -> Update of neural weight/3(W), Neural network output/2(W)
  Manual Switch/1 -> Neural network output/1(phi_net), Update of neural weight/1(phi_net)
  Hyperbolic/1(output) -> Manual Switch/1
  state/1 -> Hyperbolic/1(input), Manual Switch/2

== system MAS_CTE/Control and plant 6/LP-based controller ==
  note: Change the serial number
  note: Change the serial number
  x_i : Inport
  delta_xi : Inport  Port=2
  delta_vi : Inport  Port=3
  a_di : Inport  Port=4
  w_i_hat : Inport  Port=5
  s_i : Inport  Port=6
  Constant : Constant  Value=[0;0;0]
  Linear programming optimisation : MATLAB Function  Commented=on  TreatAsAtomicUnit=on
  Manual Switch : ManualSwitch
  Manual Switch1 : ManualSwitch  CurrentSetting=0
  Nominal Controller : MATLAB Function  TreatAsAtomicUnit=on
  Saturation : Saturate  UpperLimit=UpperLimit  LowerLimit=LowerLimit
  Scope : Scope
  Scope4 : Scope  Commented=on  NumInputPorts=2
  Subsystem : Subsystem
  u_1 : Outport
  wires:
  Nominal Controller/2(G_i) -> Subsystem/1(G_i), Linear programming optimisation/2(G_i)
  Linear programming optimisation/1(u_i) -> Manual Switch/2
  Nominal Controller/3(expect) -> Linear programming optimisation/3("expect ")
  Linear programming optimisation/2(now) -> Scope4/1
  Linear programming optimisation/3(expect) -> Scope4/2
  Nominal Controller/1(u_i) -> Subsystem/3(Nominal), Saturation/1, Manual Switch/1, Linear programming optimisation/1(u_nom)
  x_i/1 -> Nominal Controller/1(x_i)
  delta_xi/1 -> Nominal Controller/2(delta_xi)
  delta_vi/1 -> Nominal Controller/3(delta_vi)
  a_di/1 -> Nominal Controller/4(a_di)
  w_i_hat/1 -> Nominal Controller/5(u_i_hat)
  s_i/1 -> Nominal Controller/6(s_i)
  Saturation/1 -> Subsystem/2(Saturated)
  Manual Switch/1 -> u_1/1
  Subsystem/1(xi_i) -> Manual Switch1/1, Scope/1
  Constant/1 -> Manual Switch1/2
  Manual Switch1/1 -> Nominal Controller/7(xi_i)

== system MAS_CTE/Control and plant 6/Neural network ==
  esti_s : Inport
  state : Inport  Port=2
  Hyperbolic : MATLAB Function  TreatAsAtomicUnit=on
  Manual Switch : ManualSwitch
  Neural network output : MATLAB Function  TreatAsAtomicUnit=on
  Update of neural weight : MATLAB Function  TreatAsAtomicUnit=on
  Weight initialisation : MATLAB Function  TreatAsAtomicUnit=on
  Weight update : Integrator  InitialConditionSource=external
  w_i : Outport
  wires:
  Update of neural weight/1(W_dot) -> Weight update/1
  esti_s/1 -> Update of neural weight/2(esti_s)
  Neural network output/1(w_i) -> w_i/1
  Weight initialisation/1(W_0) -> Weight update/2
  Weight update/1 -> Update of neural weight/3(W), Neural network output/2(W)
  Manual Switch/1 -> Neural network output/1(phi_net), Update of neural weight/1(phi_net)
  Hyperbolic/1(output) -> Manual Switch/1
  state/1 -> Hyperbolic/1(input), Manual Switch/2

== system MAS_CTE/Self-calculation 1/Observer ==
  note: Current version:
      | NN-based sliding mode observer, the estimation includes epsilon_hat and u_hat
  note: Change the serial number
  state : Inport
  u_i : Inport  Port=2
  Bus Creator : BusCreator  Inputs=2
  Estimation sliding surface : MATLAB Function  TreatAsAtomicUnit=on
  Neural network : Subsystem
  Observer iteration : MATLAB Function  TreatAsAtomicUnit=on
  Real_E : Scope
  esti_s : Scope
  esti_x : Scope
  satu : Scope
  virtual_pos : Integrator  InitialCondition=InitialCondition  ContinuousStateAttributes='x_hat'
  virtual_vel : Integrator  InitialCondition=[0;0;0]  ContinuousStateAttributes='v_hat'
  w_i : Scope
  E_i : Outport
  wires:
  Observer iteration/3(v_hat_dot) -> virtual_vel/1
  Estimation sliding surface/3(esti_v) -> Observer iteration/6(esti_v)
  Observer iteration/1(E_i) -> E_i/1, Real_E/1
  state/1 -> Neural network/1(state), Observer iteration/1(state), Estimation sliding surface/1(state)
  Observer iteration/2(satu) -> satu/1
  virtual_vel/1 -> Bus Creator/2, virtual_pos/1
  Estimation sliding surface/1(esti_s) -> Neural network/2(esti_s), Observer iteration/4(esti_s), esti_s/1
  Estimation sliding surface/2(esti_x) -> esti_x/1, Observer iteration/5(esti_x)
  Bus Creator/1 -> Estimation sliding surface/2(state_hat)
  Neural network/1(w_i) -> w_i/1, Observer iteration/2(w_i)
  u_i/1 -> Observer iteration/3(u_i)
  virtual_pos/1 -> Bus Creator/1

== system MAS_CTE/Self-calculation 1/Tracking error calculation ==
  note: Change the serial number
  ref : Inport
  state : Inport  Port=2
  Data selection : MATLAB Function  TreatAsAtomicUnit=on
  delta_xi : Outport
  delta_vi : Outport  Port=2
  a_d : Outport  Port=3
  wires:
  state/1 -> Data selection/2(state)
  ref/1 -> Data selection/1(ref)
  Data selection/3(a_d) -> a_d/1
  Data selection/2(delta_vi) -> delta_vi/1
  Data selection/1(delta_xi) -> delta_xi/1

== system MAS_CTE/Self-calculation 2/Observer ==
  note: Change the serial number
  note: Current version:
      | NN-based sliding mode observer, the estimation includes epsilon_hat and u_hat
  state : Inport
  u_i : Inport  Port=2
  Bus Creator : BusCreator  Inputs=2
  Estimation sliding surface : MATLAB Function  TreatAsAtomicUnit=on
  Neural network : Subsystem
  Observer iteration : MATLAB Function  TreatAsAtomicUnit=on
  Real_E : Scope
  esti_s : Scope
  esti_x : Scope
  satu : Scope
  virtual_pos : Integrator  InitialCondition=InitialCondition  ContinuousStateAttributes='x_hat'
  virtual_vel : Integrator  InitialCondition=[0;0;0]  ContinuousStateAttributes='v_hat'
  w_i : Scope
  E_i : Outport
  wires:
  Observer iteration/3(v_hat_dot) -> virtual_vel/1
  Estimation sliding surface/3(esti_v) -> Observer iteration/6(esti_v)
  Observer iteration/1(E_i) -> E_i/1, Real_E/1
  state/1 -> Neural network/1(state), Observer iteration/1(state), Estimation sliding surface/1(state)
  Observer iteration/2(satu) -> satu/1
  virtual_vel/1 -> Bus Creator/2, virtual_pos/1
  Estimation sliding surface/1(esti_s) -> Neural network/2(esti_s), Observer iteration/4(esti_s), esti_s/1
  Estimation sliding surface/2(esti_x) -> esti_x/1, Observer iteration/5(esti_x)
  Bus Creator/1 -> Estimation sliding surface/2(state_hat)
  Neural network/1(w_i) -> w_i/1, Observer iteration/2(w_i)
  u_i/1 -> Observer iteration/3(u_i)
  virtual_pos/1 -> Bus Creator/1

== system MAS_CTE/Self-calculation 2/Tracking error calculation ==
  note: Change the serial number
  ref : Inport
  state : Inport  Port=2
  Data selection : MATLAB Function  TreatAsAtomicUnit=on
  delta_xi : Outport
  delta_vi : Outport  Port=2
  a_d : Outport  Port=3
  wires:
  state/1 -> Data selection/2(state)
  ref/1 -> Data selection/1(ref)
  Data selection/3(a_d) -> a_d/1
  Data selection/2(delta_vi) -> delta_vi/1
  Data selection/1(delta_xi) -> delta_xi/1

== system MAS_CTE/Self-calculation 3/Observer ==
  note: Change the serial number
  note: Current version:
      | NN-based sliding mode observer, the estimation includes epsilon_hat and u_hat
  state : Inport
  u_i : Inport  Port=2
  Bus Creator : BusCreator  Inputs=2
  Estimation sliding surface : MATLAB Function  TreatAsAtomicUnit=on
  Neural network : Subsystem
  Observer iteration : MATLAB Function  TreatAsAtomicUnit=on
  Real_E : Scope
  esti_s : Scope
  esti_x : Scope
  satu : Scope
  virtual_pos : Integrator  InitialCondition=InitialCondition  ContinuousStateAttributes='x_hat'
  virtual_vel : Integrator  InitialCondition=[0;0;0]  ContinuousStateAttributes='v_hat'
  w_i : Scope
  E_i : Outport
  wires:
  Observer iteration/3(v_hat_dot) -> virtual_vel/1
  Estimation sliding surface/3(esti_v) -> Observer iteration/6(esti_v)
  Observer iteration/1(E_i) -> E_i/1, Real_E/1
  state/1 -> Neural network/1(state), Observer iteration/1(state), Estimation sliding surface/1(state)
  Observer iteration/2(satu) -> satu/1
  virtual_vel/1 -> Bus Creator/2, virtual_pos/1
  Estimation sliding surface/1(esti_s) -> Neural network/2(esti_s), Observer iteration/4(esti_s), esti_s/1
  Estimation sliding surface/2(esti_x) -> esti_x/1, Observer iteration/5(esti_x)
  Bus Creator/1 -> Estimation sliding surface/2(state_hat)
  Neural network/1(w_i) -> w_i/1, Observer iteration/2(w_i)
  u_i/1 -> Observer iteration/3(u_i)
  virtual_pos/1 -> Bus Creator/1

== system MAS_CTE/Self-calculation 3/Tracking error calculation ==
  note: Change the serial number
  ref : Inport
  state : Inport  Port=2
  Data selection : MATLAB Function  TreatAsAtomicUnit=on
  delta_xi : Outport
  delta_vi : Outport  Port=2
  a_d : Outport  Port=3
  wires:
  state/1 -> Data selection/2(state)
  ref/1 -> Data selection/1(ref)
  Data selection/3(a_d) -> a_d/1
  Data selection/2(delta_vi) -> delta_vi/1
  Data selection/1(delta_xi) -> delta_xi/1
